simulink model "Punto_5"  (R2022a)
settings: Solver=VariableStepAuto  StartTime=0.0  StopTime=10.0  RelTol=1e-3
undefined symbols (not defined in the file): A, B
settings Model: Creator=nicoquintero  LastModifiedBy=garzo
settings SolverCC: AlgebraicLoopSolver=TrustRegion
settings DebuggingCC: UnconnectedInputMsg=warning  UnconnectedOutputMsg=warning  UnconnectedLineMsg=warning  SFMachineParentedDataDiag=warning

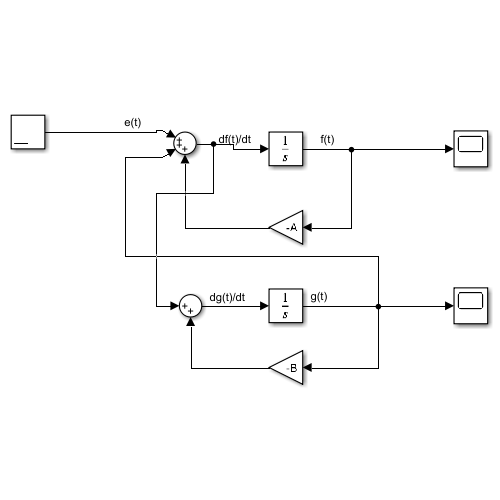
[thumbnail: Simulink's stored preview of the top-level diagram]
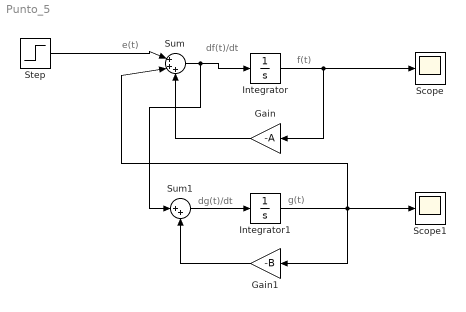
== system Punto_5 ==
  note: e(t)
  note: g(t)
  note: dg(t)/dt
  note: f(t)
  note: df(t)/dt
  Gain : Gain  Gain=-A
  Gain1 : Gain  Gain=-B
  Integrator : Integrator
  Integrator1 : Integrator
  Scope : Scope
  Scope1 : Scope
  Step : Step  SampleTime=0
  Sum : Sum  Inputs=|+++
  Sum1 : Sum  Inputs=|++
  wires:
  Integrator/1 -> Scope/1, Gain/1
  Sum/1 -> Sum1/1, Integrator/1
  Integrator1/1 -> Sum/2, Scope1/1, Gain1/1
  Gain/1 -> Sum/3
  Step/1 -> Sum/1
  Gain1/1 -> Sum1/2
  Sum1/1 -> Integrator1/1
